simulink model "gov_basics"  (R2020a)
settings: Solver=VariableStepAuto  StartTime=0.0  StopTime=10.0  RelTol=1e-3
values from neighbouring files (symbols this model uses):
  Tf = 0.5    [main.m]
  Tg = 0.1    [main.m]
  To = 0.01    [main.m]
  Tp = 0.01    [main.m]
settings Model: Creator=erlended  LastModifiedBy=erlended

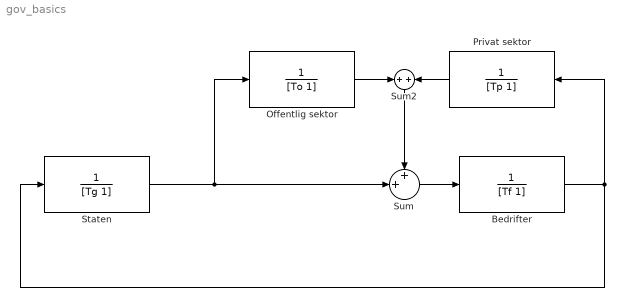
== system gov_basics ==
  Bedrifter : TransferFcn  Denominator=[Tf 1]
  Offentlig sektor : TransferFcn  Denominator=[To 1]
  Privat sektor : TransferFcn  Denominator=[Tp 1]
  Staten : TransferFcn  Denominator=[Tg 1]
  Sum : Sum  Inputs=++|
  Sum2 : Sum  Inputs=+|+
  wires:
  Offentlig sektor/1 -> Sum2/1
  Privat sektor/1 -> Sum2/2
  Sum2/1 -> Sum/1
  Bedrifter/1 -> Staten/1, Privat sektor/1
  Sum/1 -> Bedrifter/1
  Staten/1 -> Sum/2, Offentlig sektor/1
